simulink model "simulation_EKF_sonar"  (R2020a)
settings: Solver=VariableStepAuto  StartTime=0.0  StopTime=180  RelTol=1e-3
values from neighbouring files (symbols this model uses):
  distanceFromWall = 8    [missionC.m]
  nav_DT = 0.1    [initialization_nav.m]
  nav_giro = 2    [initialization_nav.m]
  nav_h0 = 0    [initialization_nav.m]
  nav_lat0 = cornerC(1)    [initialization_nav.m]
  nav_lon0 = cornerC(2)    [initialization_nav.m]
  nav_plane_AB = coefficient_plane(nav_A,nav_B)    [initialization_nav.m]
  nav_plane_BC = coefficient_plane(nav_B,nav_C)    [initialization_nav.m]
  nav_plane_CD = coefficient_plane(nav_C,nav_D)    [initialization_nav.m]
  nav_plane_DA = coefficient_plane(nav_D,nav_A)    [initialization_nav.m]
undefined symbols (not defined in the file or in its folder): nav_A, nav_B, nav_C, nav_D
(part 2 of 2)

== matlab function simulation_EKF_sonar/Navigation1/Extended Kalman Filter/MISURA VIRTUALE/MATLAB Function ==
  data: x_k_k_1 input; flag_vect input; mis_vect input; e output size=6 1; H output size=6 3; J input; nav_plane_AB parameter; nav_plane_BC parameter; nav_plane_CD parameter; nav_plane_DA parameter
%%
% chiedere ai sensoristi se le posizioni dei sensori equivalgono al centro
% di massa del robot o dobbiamo considerare spostamenti e orientazioni
% relative alla terna body
%%

function [e, H] = virtual(x_k_k_1, flag_vect, mis_vect, J, nav_plane_AB, nav_plane_BC, nav_plane_CD, nav_plane_DA)

    e = zeros(6,1);
    h = zeros(6,1);
    z = zeros(6,1);
    H = zeros(6,3);
    
    
    %valutazione misure GPS
    if mis_vect(3)==1                                   %se i dati del GPS sono validi
        if flag_vect(1) == 1 && flag_vect(2) == 1       %se i dati del GPS sono nuovi
            
            z = z + [mis_vect(1) mis_vect(2) 0 0 0 0]';
            h = h + [x_k_k_1(1)   x_k_k_1(2) 0 0 0 0]';
        
            H(1,:)= [1 0 0];
            H(2,:)= [0 1 0];
        end
    end
    
    %valutazione misure depth
    if flag_vect(4) == 1                                 %se i dati del profondimetro sono nuovi
            
        z = z + [0 0 mis_vect(4) 0 0 0]'; 
        h = h + [0 0  x_k_k_1(3) 0 0 0]';

        H(3,:)= [0 0 1];
    end
    
    %valutiamo ora le misure virtuali solo se quelle del GPS non sono
    %valide
    if mis_vect(3)==0                      %se i dati del GPS non sono validi
        
        if flag_vect(5) == 1               %se i dati del sonar di prua sono nuovi
                
                versore_son_NED = J*[1 0 0]';          %versore terna NED sonar prua
                
                [distanza, plane] = inter(x_k_k_1, versore_son_NED ,nav_plane_AB,nav_plane_BC,nav_plane_CD,nav_plane_DA);
                z = z + [0 0 0 mis_vect(5) 0 0]'; 
                h = h + [0 0 0 distanza    0 0]';
                
                H_new=zeros(1,3);
                [H_new(1), H_new(2), H_new(3)] = calc_H_vect(x_k_k_1, versore_son_NED,plane);
                H(4,:) = H_new;                
        end
    
        if flag_vect(6) == 1               %se i dati del sonar destro sono nuovi
                
                versore_son_NED = J*[0 1 0]';          %versore terna NED sonar dx
                
                [distanza, plane] = inter(x_k_k_1, versore_son_NED ,nav_plane_AB,nav_plane_BC,nav_plane_CD,nav_plane_DA);
                z = z + [0 0 0 0 mis_vect(6) 0]'; 
                h = h + [0 0 0 0 distanza    0]';
                
                H_new=zeros(1,3);
                [H_new(1), H_new(2), H_new(3)] = calc_H_vect(x_k_k_1, versore_son_NED,plane);
                H(5,:) = H_new;
        end
    
        if flag_vect(7) == 1               %se i dati del sonar sinistro sono nuovi
                 
                versore_son_NED = J*[0 -1 0]';          %versore terna NED sonar sx
                
                [distanza, plane] = inter(x_k_k_1, versore_son_NED ,nav_plane_AB,nav_plane_BC,nav_plane_CD,nav_plane_DA);
                z = z + [0 0 0 0 0 mis_vect(7)]'; 
                h = h + [0 0 0 0 0 distanza   ]'; 
                
                H_new=zeros(1,3);
                [H_new(1), H_new(2), H_new(3)] = calc_H_vect(x_k_k_1, versore_son_NED,plane);
                H(6,:) = H_new;
        end
    end
    
    e = z - h;
    
    %%riduco le dimensioni della matrice H e del vettore e
    
    i=0;
    if mis_vect(3) == 0                    %se i dati del GPS non sono validi
        H(1-i,:) = [];
        e(1-i) = [];
        i=i+1;
        H(2-i,:) = [];
        e(2-i) = [];
        i=i+1;
        if flag_vect(4) == 0               %se i dati del profondimetro non sono nuovi
            H(3-i,:) = [];
            e(3-i) = [];
            i=i+1;
        end
        if flag_vect(5) == 0               %se i dati del sonar di prua non sono nuovi
            H(4-i,:) = [];
            e(4-i) = [];
            i=i+1;
        end
        if flag_vect(6) == 0               %se i dati del sonar sinistro non sono nuovi
            H(5-i,:) = [];
            e(5-i) = [];
            i=i+1;
        end
        if flag_vect(7) == 0               %se i dati del sonar destro non sono nuovi
            H(6-i,:) = [];
            e(6-i) = [];
        end
    % da qui invece abbiamo il GPS valido
    else
        if flag_vect(1)==0 || flag_vect(2)==0  %se i dati del GPS non sono nuovi
            H(1-i,:) = [];
            e(1-i) = [];
            i=i+1;
            H(2-i,:) = [];
            e(2-i) = [];
            i=i+1;
        end
        
        if flag_vect(4) == 0               %se i dati del profondimetro non sono nuovi
            H(3-i,:) = [];
            e(3-i) = [];
            i=i+1;
        end
        
        H(4-i,:) = [];                      %annulliamo le misure dei sonar
        e(4-i) = [];
        i=i+1;
        H(5-i,:) = [];
        e(5-i) = [];
        i=i+1;
        H(6-i,:) = [];        
        e(6-i) = [];    
    end
    i=0;
end



%%
%%%%%%%%%%%%%%%%%%%%%%%%%%%%%%%%%%%%%%%%%%%%%%%%%%%%%%%%%%%%%%%%%%%%%%%%%%%%%%%%%%%%%%%%

function [dist, plane] = inter(pos, versore_son_NED,nav_plane_AB,nav_plane_BC,nav_plane_CD,nav_plane_DA)
    
    %calcolo della distanza dalla posizione ai piani delle pareti seguendo
    %la direzione data dal versore del sonar

    t_AB = -(pos(1)+nav_plane_AB(2)*pos(2)+nav_plane_AB(4))/(nav_plane_AB(2)*versore_son_NED(2)+versore_son_NED(1));
    t_BC = -(pos(1)+nav_plane_BC(2)*pos(2)+nav_plane_BC(4))/(nav_plane_BC(2)*versore_son_NED(2)+versore_son_NED(1));
    t_CD = -(pos(1)+nav_plane_CD(2)*pos(2)+nav_plane_CD(4))/(nav_plane_CD(2)*versore_son_NED(2)+versore_son_NED(1));
    t_DA = -(pos(1)+nav_plane_DA(2)*pos(2)+nav_plane_DA(4))/(nav_plane_DA(2)*versore_son_NED(2)+versore_son_NED(1));
    
    if t_AB < 0
        t_AB = inf;
    end
    if t_BC < 0
        t_BC = inf;
    end
    if t_CD < 0
        t_CD = inf;
    end
    if t_DA < 0
        t_DA = inf;
    end
           
    [dist, index] = min([t_AB t_BC t_CD t_DA]);
    dist = dist - 0.267;       %va tolto il raggio del robot rispetto al centro di massa
    
    switch index
        case 1
            plane = nav_plane_AB;
        case 2
            plane = nav_plane_BC;
        case 3
            plane = nav_plane_CD;
        case 4
            plane = nav_plane_DA;
        otherwise
            plane=[0 0 0 0];
            disp('errore nella intersezione del piano')
    end
    
end

function [H1, H2, H3]= calc_H_vect(pos, sonar, plane)

    H1 = sign(pos(1) + plane(4) + pos(2)*plane(2))/abs(sonar(1) + plane(2)*sonar(2));
    H2 = (plane(2)*sign(pos(1) + plane(4) + pos(2)*plane(2)))/abs(sonar(1) + plane(2)*sonar(2));   
    H3 = 0;
end

== matlab function simulation_EKF_sonar/Navigation1/Calcolo distaza pareti/Calcolo distanza dalle pareti ==
  data: pos_es input; dpp output; dps output; parete_attuale input; nav_plane_AB parameter; nav_plane_BC parameter; nav_plane_CD parameter; nav_plane_DA parameter; nav_giro parameter
% Applicando la formula della distanza di un punto da un piano ottengo la
% distanza della posizione dell'AUV dalla parete d'interesse. 

function [dpp,dps] = dpp_dps_calculator(pos_es, parete_attuale, nav_plane_AB, nav_plane_BC, nav_plane_CD, nav_plane_DA, nav_giro)
    
%selezione della parete di pattugliamento e successiva
    switch parete_attuale
        
        case 1
           coef = nav_plane_AB;            %parete attuale AB
           if nav_giro == 1
               coef_succ = nav_plane_BC;   %parete succ BC
           else
               coef_succ = nav_plane_DA;   %parete succ DA
           end
           
        case 2
           coef = nav_plane_BC;            %parete attuale BC
           if nav_giro == 1
               coef_succ = nav_plane_CD;   %parete succ CD
           else
               coef_succ = nav_plane_AB;   %parete succ AB
           end
           
        case 3
           coef = nav_plane_CD;            %parete attuale CD
           if nav_giro == 1
               coef_succ = nav_plane_DA;   %parete succ DA
           else
               coef_succ = nav_plane_BC;   %parete succ BC
           end
        case 4
           coef = nav_plane_DA;            %parete attuale DA
           if nav_giro == 1
               coef_succ = nav_plane_AB;   %parete succ AB
           else
               coef_succ = nav_plane_CD;   %parete succ CD
           end
        otherwise
            coef = [0 0 0 0];
            coef_succ = [0 0 0 0];
    end

    dpp = abs(coef(1)*pos_es(1)+coef(2)*pos_es(2)-coef(3)*pos_es(3)+coef(4))/norm([coef(1) coef(2) coef(3)]);
    dps = abs(coef_succ(1)*pos_es(1)+coef_succ(2)*pos_es(2)-coef_succ(3)*pos_es(3)+coef_succ(4))/norm([coef_succ(1) coef_succ(2) coef_succ(3)]);
   
end

== matlab function simulation_EKF_sonar/Navigation1/Extended Kalman Filter/PREDIZIONE/Passo di Predizione ==
  data: x0 input; P0 input; x_k_1 input; u_k_1 input; x_k output; P_k_1 input; P_k output size=3 3; J input; L input; Q_k_1 input; nav_DT parameter; nav_flag_init input; nav_flag_init output
%% Passo di PREDIZIONE

function [x_k,  P_k, nav_flag_init] = prediction(x0, P0, x_k_1, u_k_1,  P_k_1, J, L, Q_k_1, nav_DT, nav_flag_init)
    
    x_k = zeros(3,1);
    P_k = zeros(3,3);

    % il valore di nav_flag_init è all'inizio della simulazione pari a 0
    % appena c'è il primo dato disponibile del GPS (insieme al profondimetro)
    % si assume quella come punto di inizializzazione del filtro.

    if nav_flag_init ~= 0      
        if nav_flag_init == 1
            x_k_1 = x0;
            P_k_1 = P0;
            nav_flag_init = 2;      % =2 così l'inizializzazione è fatta una sola volta.
        end
        
        %passo di predizione       
        x_k = x_k_1 + nav_DT*J*u_k_1;
        P_k = P_k_1 + L*Q_k_1*L';               %la matrice F è F = I
           
    end
end

== matlab function simulation_EKF_sonar/Navigation1/Extended Kalman Filter/Subsystem/MATLAB Function4 ==
  data: flag_DVL output; DVL_new input; DVL_now output; DVL_old input
function [flag_DVL, DVL_now] = fcn(DVL_new, DVL_old)

    if isnan(DVL_new(1,1)) || isnan(DVL_new(2,1)) || isnan(DVL_new(3,1))
        DVL_now = DVL_old;
        flag_DVL = 1;
        disp('Misura DVL non valida')
    else
        DVL_now = DVL_new;
        flag_DVL = 0;
    end  
end

== matlab function simulation_EKF_sonar/Navigation1/Extended Kalman Filter/Subsystem1/MATLAB Function4 ==
  data: flag_AHRS output; AHRS_new input; AHRS_now output; AHRS_old input
function [flag_AHRS, AHRS_now] = fcn(AHRS_new, AHRS_old)

    if isnan(AHRS_new(1,1)) || isnan(AHRS_new(2,1)) || isnan(AHRS_new(3,1))
        AHRS_now = AHRS_old;
        flag_AHRS = 1;
        disp('Misura AHRS non valida')
    else
        AHRS_now = AHRS_new;
        flag_AHRS = 0;
    end  
end

== matlab function simulation_EKF_sonar/Navigation1/Extended Kalman Filter/Subsystem2/MATLAB Function4 ==
  data: Q input; Q_k_1 input; Q_k output; flag_AHRS input; flag_DVL input
function Q_k = fcn(Q, Q_k_1, flag_AHRS, flag_DVL)

    Q_k = Q;
    
    K=10;
    if flag_DVL == 1
       Q_k = Q_k_1 + K*diag([0,0,0,(0.012)^2,(0.012)^2,(0.012)^2]);
    end
    
    if flag_AHRS == 1
       Q_k = Q_k_1 + K*diag([0.0087, 0.0087, 0.0017,0,0,0]);  
    end
        
end

== matlab function simulation_EKF_sonar/Navigation1/MATLAB Function ==
  data: u input; y output
function y = Wrap2pi(u)
y = [0;0;0];
coder.extrinsic('wrapToPi');
y = wrapToPi(u);
end

== matlab function simulation_EKF_sonar/Navigation1/NED2ECEF ==
  data: pos_es_NED input; pos_es_ECEF output; nav_lat0 parameter; nav_lon0 parameter; nav_h0 parameter


function pos_es_ECEF = pos_NED2ECEF(pos_es_NED,nav_lat0, nav_lon0, nav_h0)
     
    coder.extrinsic('evalin', 'wgs84Ellipsoid', 'ned2geodetic');
    pos_es_ECEF = zeros(3,1);
    depth = pos_es_NED(3); 
    
    [pos_es_ECEF(1),pos_es_ECEF(2),pos_es_ECEF(3)]= ned2geodetic(pos_es_NED(1),pos_es_NED(2),0,nav_lat0,nav_lon0,nav_h0,wgs84Ellipsoid);
    pos_es_ECEF(3) = depth;
end

== matlab function simulation_EKF_sonar/Navigation1/SOS/MATLAB Function ==
  data: P_es input; SOS output; DVL input; AHRS input; gyro input; contatore input size=3 1; contatore output
%% Generazione flag di emergenza
% 1. Assenza di segnali dai sensori per un determinato tempo

function [SOS, contatore] = SOS_flag(P_es, DVL, AHRS, gyro, contatore)
    SOS=0;
 
    soglia_P = 10; %[m^2]
    if P_es(1,1)+P_es(2,2) > soglia_P || P_es(3,3) > soglia_P
        SOS=1;
    end
    
    if DVL == 1 
        contatore(1) = contatore(1) + 1;
    else
        contatore(1) = 0;
    end
    
    if AHRS == 1 
        contatore(2) = contatore(2) + 1;
    else
        contatore(2) = 0;
    end
    
    if gyro == 1 
        contatore(3) = contatore(3) + 1;
    else
        contatore(3) = 0;
    end
    
    if max(contatore) > 20
        SOS=1;
    end
    
    

end

== matlab function simulation_EKF_sonar/Navigation1/Subsystem1/MATLAB Function4 ==
  data: flag_gyro output; gyro_new input; gyro_now output; gyro_old input
function [flag_gyro, gyro_now] = fcn(gyro_new, gyro_old)

    if isnan(gyro_new(1,1)) || isnan(gyro_new(2,1)) || isnan(gyro_new(3,1))
        gyro_now = gyro_old;
        flag_gyro = 1;
        disp('Misura gyro non valida')
    else
        gyro_now = gyro_new;
        flag_gyro = 0;
    end  
end

== matlab function simulation_EKF_sonar/Navigation1/Calcolo distaza pareti/Calcolo orientazione dalla parete ==
  data: pos_es input; orient_parete output; parete_attuale input; orient input; nav_plane_AB parameter; nav_plane_BC parameter; nav_plane_CD parameter; nav_plane_DA parameter
function orient_parete  = orient_parete_calculator(pos_es, parete_attuale, orient, nav_plane_AB, nav_plane_BC, nav_plane_CD, nav_plane_DA)
    
    %consideriamo angoli di pitch e roll nulli, cioè calcoliamo
    %l'orientazione rispetto alla parete solo considerando rotazioni di yaw
    %(piano xy)

    Yaw   = orient(3);
    R_z = [cos(Yaw)     sin(Yaw)       0     ;
           -sin(Yaw)    cos(Yaw)       0     ;
              0            0           1    ];
    v_pos= R_z'*[1 0 0]';  %versore della retta lungo l'asse x (in body) in NED,
                       %cioè la direzione di riferimento di prua del veicolo     
    
    %selezione della parete di pattugliamento
switch parete_attuale                      
    case 1
        %% Piano di pattugliamento AB
        versore_plane_NED = [nav_plane_AB(1) nav_plane_AB(2) 0]';    %versore normale al piano
        versore_plane_NED = versore_plane_NED/norm(versore_plane_NED);

        %calcolo distanza e intersezione lungo la normale al piano
        t_ = -(pos_es(1)+nav_plane_AB(2)*pos_es(2)+nav_plane_AB(4))/(nav_plane_AB(2)*versore_plane_NED(2)+versore_plane_NED(1));
        inter_perp=zeros(3,1);
        inter_perp(1) = pos_es(1) + versore_plane_NED(1)*t_;
        inter_perp(2) = pos_es(2) + versore_plane_NED(2)*t_;
        inter_perp(3) = pos_es(3) + versore_plane_NED(3)*t_;
        
        %calcolo distanza e intersezione lungo la direzione di prua
        t_ = -(pos_es(1)+nav_plane_AB(2)*pos_es(2)+nav_plane_AB(4))/(nav_plane_AB(2)*v_pos(2)+v_pos(1));
        inter_prua=zeros(3,1);
        inter_prua(1) = pos_es(1) + v_pos(1)*t_;
        inter_prua(2) = pos_es(2) + v_pos(2)*t_;
        inter_prua(3) = pos_es(3) + v_pos(3)*t_;
        
        coef = nav_plane_AB;
        coef(4)=[];
        orient_parete = rad2deg(asin(abs(coef*v_pos)/(norm(coef)*norm(v_pos))));
        %se orient_parete è positiva, allora ci troviamo tra - 90 e + 90 rispetto alla normale della parete 
        if t_ > 0              
            if inter_prua(1) > inter_perp(1) && inter_prua(2) < inter_perp(2)
                orient_parete = orient_parete - 90;
            else
                orient_parete = -(orient_parete - 90);
            end
        else
            if inter_prua(1) > inter_perp(1) && inter_prua(2) < inter_perp(2)
                orient_parete = (orient_parete + 90);
            else
                orient_parete = -(orient_parete + 90);
            end
        end    
    case 2
        %% Piano di pattugliamento BC
      	versore_plane_NED = [nav_plane_BC(1) nav_plane_BC(2) 0]';    %versore normale al piano
        versore_plane_NED = versore_plane_NED/norm(versore_plane_NED);

        %calcolo distanza e intersezione lungo la normale al piano
        t_ = -(pos_es(1)+nav_plane_BC(2)*pos_es(2)+nav_plane_BC(4))/(nav_plane_BC(2)*versore_plane_NED(2)+versore_plane_NED(1));
        inter_perp=zeros(3,1);
        inter_perp(1) = pos_es(1) + versore_plane_NED(1)*t_;
        inter_perp(2) = pos_es(2) + versore_plane_NED(2)*t_;
        inter_perp(3) = pos_es(3) + versore_plane_NED(3)*t_;

        %calcolo distanza e intersezione lungo la direzione di prua
        t_ = -(pos_es(1)+nav_plane_BC(2)*pos_es(2)+nav_plane_BC(4))/(nav_plane_BC(2)*v_pos(2)+v_pos(1));
        inter_prua=zeros(3,1);
        inter_prua(1) = pos_es(1) + v_pos(1)*t_;
        inter_prua(2) = pos_es(2) + v_pos(2)*t_;
        inter_prua(3) = pos_es(3) + v_pos(3)*t_;
        
        coef = nav_plane_BC;
        coef(4)=[];
        v_pos=-v_pos;
        orient_parete = rad2deg(asin(abs(coef*v_pos)/(norm(coef)*norm(v_pos))));
        %se orient_parete è positiva, allora ci troviamo tra - 90 e + 90 rispetto alla normale della parete 
        if t_ > 0              
            if inter_prua(1) > inter_perp(1) && inter_prua(2) > inter_perp(2)
                orient_parete = orient_parete - 90;
            else
                orient_parete = -(orient_parete - 90);
            end
        else
            if inter_prua(1) > inter_perp(1) && inter_prua(2) > inter_perp(2)
                orient_parete = orient_parete + 90;
            else
                orient_parete = -(orient_parete + 90);
            end
        end
        
    case 3
        %% Piano di pattugliamento CD
      	versore_plane_NED = [nav_plane_CD(1) nav_plane_CD(2) 0]';    %versore normale al piano
        versore_plane_NED = versore_plane_NED/norm(versore_plane_NED);

        %calcolo distanza e intersezione lungo la normale al piano
        t_ = -(pos_es(1)+nav_plane_CD(2)*pos_es(2)+nav_plane_CD(4))/(nav_plane_CD(2)*versore_plane_NED(2)+versore_plane_NED(1));
        inter_perp=zeros(3,1);
        inter_perp(1) = pos_es(1) + versore_plane_NED(1)*t_;
        inter_perp(2) = pos_es(2) + versore_plane_NED(2)*t_;
        inter_perp(3) = pos_es(3) + versore_plane_NED(3)*t_;

        %calcolo distanza e intersezione lungo la direzione di prua
        t_ = -(pos_es(1)+nav_plane_CD(2)*pos_es(2)+nav_plane_CD(4))/(nav_plane_CD(2)*v_pos(2)+v_pos(1));
        inter_prua=zeros(3,1);
        inter_prua(1) = pos_es(1) + v_pos(1)*t_;
        inter_prua(2) = pos_es(2) + v_pos(2)*t_;
        inter_prua(3) = pos_es(3) + v_pos(3)*t_;
        
        coef = nav_plane_CD;
        coef(4)=[];
        v_pos=-v_pos;
        orient_parete = rad2deg(asin(abs(coef*v_pos)/(norm(coef)*norm(v_pos))));
        %se orient_parete è positiva, allora ci troviamo tra - 90 e + 90 rispetto alla normale della parete 
        if t_ > 0              
            if inter_prua(1) > inter_perp(1) && inter_prua(2) < inter_perp(2)
                orient_parete = -orient_parete + 90;
            else
                orient_parete = orient_parete - 90;
            end
        else
             if inter_prua(1) > inter_perp(1) && inter_prua(2) < inter_perp(2)
                orient_parete = -orient_parete - 90;
            else
                orient_parete = orient_parete + 90;
            end
        end
        
    case 4
        %% Piano di pattugliamento DA
      	versore_plane_NED = [nav_plane_DA(1) nav_plane_DA(2) 0]';    %versore normale al piano
        versore_plane_NED = versore_plane_NED/norm(versore_plane_NED);

        %calcolo distanza e intersezione lungo la normale al piano
        t_ = -(pos_es(1)+nav_plane_DA(2)*pos_es(2)+nav_plane_DA(4))/(nav_plane_DA(2)*versore_plane_NED(2)+versore_plane_NED(1));
        inter_perp=zeros(3,1);
        inter_perp(1) = pos_es(1) + versore_plane_NED(1)*t_;
        inter_perp(2) = pos_es(2) + versore_plane_NED(2)*t_;
        inter_perp(3) = pos_es(3) + versore_plane_NED(3)*t_;

        %calcolo distanza e intersezione lungo la direzione di prua
        t_ = -(pos_es(1)+nav_plane_DA(2)*pos_es(2)+nav_plane_DA(4))/(nav_plane_DA(2)*v_pos(2)+v_pos(1));
        inter_prua=zeros(3,1);
        inter_prua(1) = pos_es(1) + v_pos(1)*t_;
        inter_prua(2) = pos_es(2) + v_pos(2)*t_;
        inter_prua(3) = pos_es(3) + v_pos(3)*t_;
        
        coef = nav_plane_DA;
        coef(4)=[];
        orient_parete = rad2deg(asin(abs(coef*v_pos)/(norm(coef)*norm(v_pos))));
        %se orient_parete è positiva, allora ci troviamo tra - 90 e + 90 rispetto alla normale della parete 
        if t_ > 0              
            if inter_prua(1) < inter_perp(1) && inter_prua(2) < inter_perp(2)
                orient_parete = orient_parete - 90;
            else
                orient_parete = -orient_parete + 90;
            end
        else
            if inter_prua(1) < inter_perp(1) && inter_prua(2) < inter_perp(2)
                orient_parete = orient_parete + 90;
            else
                orient_parete = -orient_parete - 90;
            end
        end
        
    otherwise
        %%
       coef=[0 0 0 0];
       orient_parete = NaN;
       disp('errore nella scelta del piano')
end
    
    
end

== matlab function simulation_EKF_sonar/Navigation1/ECEF2NED ==
  data: GPS_ECEF input; GPS_NED output; nav_lat0 parameter; nav_lon0 parameter; nav_h0 parameter
%Componente di ingresso in terna ECEF
%Lat  [gradi]
%Long  [gradi]
%flag data_valid

function GPS_NED = GPS_conv_valid(GPS_ECEF, nav_lat0, nav_lon0, nav_h0)
    
    coder.extrinsic('evalin', 'wgs84Ellipsoid', 'geodetic2ned');

    if GPS_ECEF(3)==1
        GPS_NED = zeros(3,1);
        [GPS_NED(1),GPS_NED(2),GPS_NED(3)]= geodetic2ned(GPS_ECEF(1),GPS_ECEF(2),0,nav_lat0,nav_lon0,nav_h0,wgs84Ellipsoid);
        GPS_NED(3) = GPS_ECEF(3);
    else                            %qui ci risparmiamo la conversione se il dato non è valido
        GPS_NED = GPS_ECEF; 
    end
end

== matlab function simulation_EKF_sonar/Navigation1/Extended Kalman Filter/CORREZIONE/MATLAB Function ==
  data: x_k_k_1 input; x_k output; P_k_k_1 input; e input size=6 1; H input size=6 3; R_k input size=6 6; P_k output; nav_flag_init input


function [x_k, P_k] = correction(x_k_k_1,P_k_k_1, e, H, R_k,nav_flag_init)
    
     x_k = zeros(3,1);
     P_k = zeros(3,3);
     
     
    if nav_flag_init ~= 0
        %matrice ottenuta da derivata di funzione h (6x1) per i rumori sei vari
        %sensori, che sono 6. (ha dimensione 6x6)
        %andrebbero anche considerati i rumori legati all'AHRS che al momento
        %sono trascurati
        %M = eye(6,6);              %M è l'dientità
        S_k = H*P_k_k_1*H'+ R_k;
        K_k = P_k_k_1*H'*(inv(S_k));

        P_k = (eye(3)-(K_k*H))*P_k_k_1;
        x_k = x_k_k_1 + K_k * e;
    end

end

== matlab function simulation_EKF_sonar/Subsystem/Environment ==
  data: plane_AB output; plane_BC output; plane_CD output; plane_DA output
function [plane_AB,plane_BC,plane_CD,plane_DA] = fcn()
%% Inizializzazione
% Coordinate degli spigoli del bacino in lat e long fornite dal file
% missionC.m
A= zeros(1,3);
B= zeros(1,3);
C= zeros(1,3);
D= zeros(1,3);
cornerA = [43.781381; 11.282793]; % Lat/Lon [decimal degrees]      
cornerB = [43.780975; 11.283505]; % Lat/Lon [decimal degrees]       
cornerC = [43.780189; 11.282698]; % Lat/Lon [decimal degrees]       
cornerD = [43.780602; 11.281956]; % Lat/Lon [decimal degrees]

% Definizione terna NED con origine (lat0,long0,h0) coincidente al 
% cornerD
coder.extrinsic('evalin', 'wgs84Ellipsoid', 'geodetic2ned');
lat0 = cornerC(1);
lon0 = cornerC(2);
h0 = 0;

%% Conversione ECEF to NED
[A(1),A(2),A(3)] = geodetic2ned(cornerA(1),cornerA(2),0,lat0,lon0,h0,wgs84Ellipsoid);
[B(1),B(2),B(3)] = geodetic2ned(cornerB(1),cornerB(2),0,lat0,lon0,h0,wgs84Ellipsoid);
[C(1),C(2),C(3)] = geodetic2ned(cornerC(1),cornerC(2),0,lat0,lon0,h0,wgs84Ellipsoid);
[D(1),D(2),D(3)] = geodetic2ned(cornerD(1),cornerD(2),0,lat0,lon0,h0,wgs84Ellipsoid);

%% Calcolo delle distanze dalle pareti
% L'equazione del piano corrisponde a quella della retta perché il piano
% delle pareti è verticale, per cui si risolve un sistema lineare:
% l'equazione del piano deve soddisfare il passaggio da due punti.
% Il parametro a è libero, lo poniamo a=1, il parametro c relativo all'asse
% z sarà sempre pari a zero.

% questo è il sistema da risolvere
b = - (B(1)- A(1)) /( B(2) - A(2) );   %AB
d = - A(1) - A(2)*b;

e = - (C(1)-B(1))/(C(2)-B(2));         %BC
f = - B(1) - B(2)*e;

g = - (D(1) - C(1)) / (D(2) - C(2));   %CD
h = - C(1) - C(2)*g;

i = - (A(1) - D(1))/(A(2) - D(2));     %DA
l = -D(1) - D(2)*i;

% syms b d;
% [b d] = solve(A(1)+b*A(2)+d,B(1)+b*B(2)+d,b,d);
a_AB = 1;
b_AB = double(b);
c_AB = 0;
d_AB = double(d);
% 
% syms b d ;
% [b d] = solve(B(1)+b*B(2)+d,C(1)+b*C(2)+d,b,d);
a_BC = 1;
b_BC = double(e);
c_BC = 0;
d_BC = double(f);

a_CD = 1;
b_CD = double(g);
c_CD = 0;
d_CD = double(h);

a_DA = 1;
b_DA = double(i);
c_DA = 0;
d_DA = double(l);


% calcolo dei coefficienti del piano direttamente con la formula esplicita
plane_AB = [a_AB b_AB c_AB d_AB];
plane_BC = [a_BC b_BC c_BC d_BC];
plane_CD = [a_CD b_CD c_CD d_CD];
plane_DA = [a_DA b_DA c_DA d_DA];

== matlab function simulation_EKF_sonar/Navigation1/Extended Kalman Filter/Creazione vettore delle misure ==
  data: flag_vect output; GPS input; mis_vect output; depth input; s_pr input; s_dx input; s_sx input; mis_vect_prec input; J input; pos input; nav_plane_AB parameter; nav_plane_BC parameter; nav_plane_CD parameter; nav_plane_DA parameter; nav_A parameter; nav_B parameter; nav_C parameter; nav_D parameter; distanceFromWall parameter
%%
% Questa funzione impila le informazioni derivanti dai vari sensori in un
% unico vettore mis_vect 7x1.                                 
% Ci sarà un corrispondente vettore flag_vect 7x1 di flag che sarà pari a:

% flag(i) = 0  se la misura è uguale a quella arrivata nell'istante
% predecente, in tal caso la correzione non verrà effettuata
% flag(i) = 1 se la misura è stata aggiornata rispetto a quella precendente
 
% NB il controllo sulla validità dei dati del GPS è valutata nel blocco
% sucessivo

function [flag_vect,mis_vect] = misure_vector(GPS,depth,s_pr,s_dx,s_sx, mis_vect_prec,...
          J,pos, nav_plane_AB, nav_plane_BC, nav_plane_CD, nav_plane_DA, nav_A, nav_B, nav_C, nav_D, distanceFromWall)
    
    mis_vect = zeros(7,1);
    flag_vect = zeros(7,1);
	mis_vect = [GPS(1) GPS(2) GPS(3) depth s_pr s_dx s_sx]';
    
    for i=[1:7]
        if mis_vect(i) ~= mis_vect_prec(i)
            flag_vect(i) = 1;
        end
    end
    
    %valutiamo se la misura del profondimetro è valida
    if isnan(depth)  
        flag_vect(4) = 0;
    end
     
    %se i dati dei sonar qui sono utilizzabili, dobbiamo assicurarci che il 
    %loro raggio non punti verso uno spigolo, in quel caso potrebbe
    %causare una correzione errata
    
    if flag_vect(5) == 1               %se i dati del sonar di prua sono nuovi
            versore_son_NED = J*[1 0 0]';          %versore terna NED sonar prua
            flag_vect(5) = inter(pos, versore_son_NED ,nav_plane_AB,nav_plane_BC,nav_plane_CD,nav_plane_DA, nav_A, nav_B, nav_C, nav_D);       
    end

    if flag_vect(6) == 1               %se i dati del sonar destro sono nuovi
            versore_son_NED = J*[0 1 0]';          %versore terna NED sonar dx

            flag_vect(6) = inter(pos, versore_son_NED ,nav_plane_AB,nav_plane_BC,nav_plane_CD,nav_plane_DA, nav_A, nav_B, nav_C, nav_D);       
    end
    if flag_vect(7) == 1               %se i dati del sonar sinistro sono nuovi
            versore_son_NED = J*[0 -1 0]';          %versore terna NED sonar sx
            flag_vect(7) = inter(pos, versore_son_NED ,nav_plane_AB,nav_plane_BC,nav_plane_CD,nav_plane_DA, nav_A, nav_B, nav_C, nav_D);
    end 
    %la terza componente di flag_vect non sarà utilizzata. per assicurarci
    %che i dati del GPS siano validi ci rifaremo sempre su mis_vect
    
    
    
    %se il valore del sonar è NaN, non dobbiamo considerare valide le
    %misure, e se il robot troppo lontane dalle pareti
    soglia_distanza=distanceFromWall*4;
    soglia_variazione=0.8;
    if isnan(s_pr) || mis_vect(5) > soglia_distanza || abs(mis_vect(5)- mis_vect_prec(5)) > soglia_variazione
        flag_vect(5) = 0;
    end
    if isnan(s_dx) || mis_vect(6) > soglia_distanza || abs(mis_vect(6)- mis_vect_prec(6)) > soglia_variazione
        flag_vect(6) = 0;
    end
    if isnan(s_sx) || mis_vect(7) > soglia_distanza || abs(mis_vect(7)- mis_vect_prec(7)) > soglia_variazione
        flag_vect(7) = 0;
    end
end




function [flag] = inter(pos, versore_son_NED,nav_plane_AB,nav_plane_BC,nav_plane_CD,nav_plane_DA, nav_A, nav_B, nav_C, nav_D)
    
    %calcolo della distanza dalla posizione ai piani delle pareti seguendo
    %la direzione data dal versore del sonar

    t_AB = -(pos(1)+nav_plane_AB(2)*pos(2)+nav_plane_AB(4))/(nav_plane_AB(2)*versore_son_NED(2)+versore_son_NED(1));
    t_BC = -(pos(1)+nav_plane_BC(2)*pos(2)+nav_plane_BC(4))/(nav_plane_BC(2)*versore_son_NED(2)+versore_son_NED(1));
    t_CD = -(pos(1)+nav_plane_CD(2)*pos(2)+nav_plane_CD(4))/(nav_plane_CD(2)*versore_son_NED(2)+versore_son_NED(1));
    t_DA = -(pos(1)+nav_plane_DA(2)*pos(2)+nav_plane_DA(4))/(nav_plane_DA(2)*versore_son_NED(2)+versore_son_NED(1));
    
    if t_AB < 0
        t_AB = inf;
    end
    if t_BC < 0
        t_BC = inf;
    end
    if t_CD < 0
        t_CD = inf;
    end
    if t_DA < 0
        t_DA = inf;
    end
           
    [dist, index] = min([t_AB t_BC t_CD t_DA]);
    dist = dist - 0.267;       %va tolto il raggio del robot rispetto al centro di massa
    
    int=zeros(1,3);
    %calcolo l'intersezione
    int(1) = pos(1) + versore_son_NED(1)*dist;
    int(2) = pos(2) + versore_son_NED(2)*dist;
    int(3) = 0;
    
    
    
    soglia_spigolo = 5;          %distanza massima dallo spigolo entro la quale 
                       %la misura del sonar non è buona
    flag=1;
    switch index
        case 1      
            if norm(int-nav_A) < soglia_spigolo || norm(int-nav_B) < soglia_spigolo
                flag=0;
            end
        case 2
            if norm(int-nav_B) < soglia_spigolo || norm(int-nav_C) < soglia_spigolo
                flag=0;
            end
        case 3
            if norm(int-nav_C) < soglia_spigolo || norm(int-nav_D) < soglia_spigolo
                flag=0;
            end
        case 4
            if norm(int-nav_D) < soglia_spigolo || norm(int-nav_A) < soglia_spigolo
                flag=0;
            end
        otherwise
            disp('errore nella intersezione del piano')
    end
end
